simulink model "testLidarSensorPlacement"  (R2024a)
settings: Solver=VariableStepAuto  StartTime=0.0  StopTime=inf  RelTol=1e-3
settings Model: Creator=ckammer  LastModifiedBy=ckammer

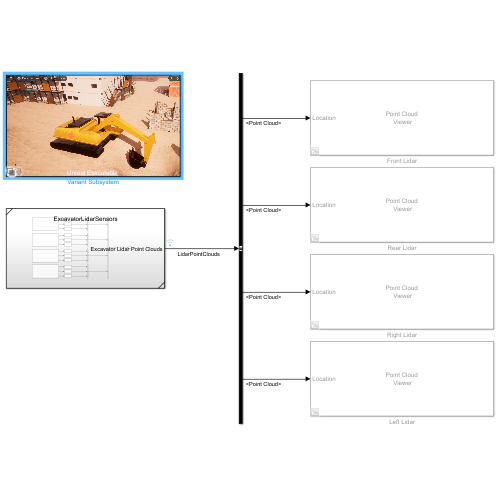
[thumbnail: Simulink's stored preview of the top-level diagram]
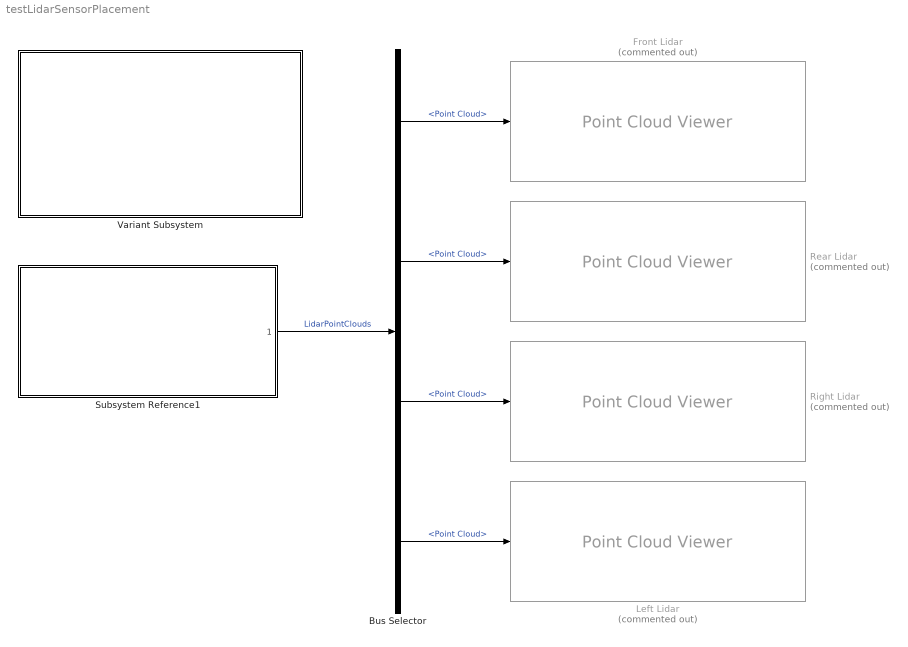
== system testLidarSensorPlacement ==
  Bus Selector : BusSelector  OutputSignals=Front Lidar.Point Cloud,Rear Lidar.Point Cloud,Right Lidar.Point Cloud,Left Lidar.Point Cloud
  Front Lidar : PointCloudViewer  Commented=on  FigPos=[1 910 1536 836.8]
  Left Lidar : PointCloudViewer  Commented=on  FigPos=[1 910 1536 836.8]
  Rear Lidar : PointCloudViewer  Commented=on  FigPos=[1 910 1536 836.8]
  Right Lidar : PointCloudViewer  Commented=on  FigPos=[1 910 1536 836.8]
  Subsystem Reference1 : Subsystem  ReferencedSubsystem=ExcavatorLidarSensors
  Variant Subsystem : Subsystem  Variant=on  VariantChoicesSpecifier={'ExcavatorUnrealExecutableSceneConfiguration', 'ExcavatorUnrealEditorSceneConfiguration'}  VariantChoicesEnumeration=myEnum  VariantControlVariable=myVCV  VariantControlMode=label  LabelModeActiveChoice=ExcavatorUnrealExecutableSceneConfiguration  mask{UnrealSceneSource=Unreal Executable}
      mask prompts: UnrealSceneSource "Unreal Scene Source Selection"
  wires:
  Subsystem Reference1/1 -> Bus Selector/1  "LidarPointClouds"
  Bus Selector/1 -> Front Lidar/1  "<Point Cloud>"
  Bus Selector/2 -> Rear Lidar/1  "<Point Cloud>"
  Bus Selector/3 -> Right Lidar/1  "<Point Cloud>"
  Bus Selector/4 -> Left Lidar/1  "<Point Cloud>"

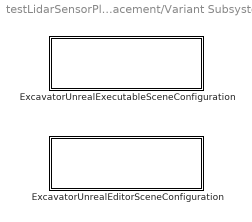
== system testLidarSensorPlacement/Variant Subsystem ==
  ExcavatorUnrealEditorSceneConfiguration : Subsystem  VariantControl=ExcavatorUnrealEditorSceneConfiguration  ReferencedSubsystem=ExcavatorUnrealEditorSceneConfiguration
  ExcavatorUnrealExecutableSceneConfiguration : Subsystem  VariantControl=ExcavatorUnrealExecutableSceneConfiguration  ReferencedSubsystem=ExcavatorUnrealExecutableSceneConfiguration
